simulink model "SIL_block"  (R2021b)
settings: Solver=FixedStepAuto  StartTime=0.0  StopTime=5  FixedStep=0.07  RelTol=1e-3
libraries: pil_lib x1
settings Model: Creator=Admin  LastModifiedBy=Admin
settings SolverCC: AlgebraicLoopSolver=TrustRegion
settings OptimizationCC: DefaultParameterBehavior=Inlined  EnhancedBackFolding=on  PassReuseOutputArgsThreshold=0  OptimizeBlockOrder=speed  DifferentSizesBufferReuse=on  OptimizationCustomize=off
settings DebuggingCC: ParameterTunabilityLossMsg=error  SFUnexpectedBacktrackingDiag=warning  SFNoUnconditionalDefaultTransitionDiag=warning  SFMachineParentedDataDiag=warning
settings SFSimCC: MATLABDynamicMemAlloc=off
settings RTWCC: GenCodeOnly=on  GenerateReport=on  BuildConfiguration=Debug  LaunchReport=on  CheckMdlBeforeBuild=Warning
settings CodeAppCC: ForceParamTrailComments=on  OperatorAnnotations=on  EnableCustomComments=on
settings ConfigComp: CovEnable=on  CovScope=Subsystem  RecordCoverage=on  CovPath=Subsystem/PID Controller1  CovMetricSettings=we  PLC_TargetIDE=codesys23  PLC_MultiTBSigbuilderTimeRange=off  PLC_InlineEnumCastFunction=off

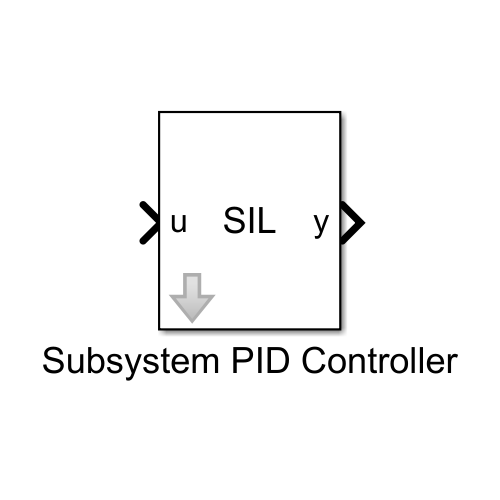
[thumbnail: Simulink's stored preview of the top-level diagram]
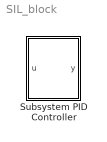
== system SIL_block ==
  Subsystem PID Controller : Subsystem  DialogController=pil_create_dialog  LoadFcn=|
      | try
      |    if ~strcmp(rtw.pil.getPILVersion, '9.11 (R2021b)_15')
      |       set_param(gcb, 'DialogController', '');
      |       set_param(gcb, 'DialogControllerArgs', '');
      |    end
      | catch e
      |       set_param(gcb, 'DialogController', '');
      |       set_param(gcb, 'DialogControllerArgs', '');
      | end
      mask help: PIL:pil:XILBlockMaskDesc
      mask Display: disp('SIL');

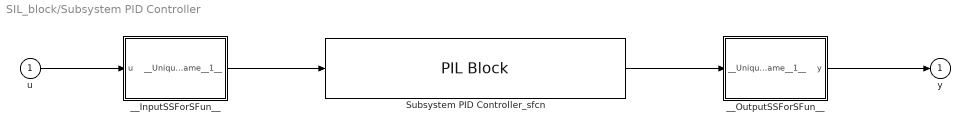
== system SIL_block/Subsystem PID Controller ==
  u : Inport
  Subsystem PID Controller_sfcn : pil_lib/PIL Block  SimulationMode=SIL  IsTopModelPIL=off  CodeDir=Subsystem_ert_rtw  AnchorDir=C:\Users\Admin\Documents\OneDrive\Рабочий стол\ПСвСМ 2022\Лекция1_23_PROGRAM  ConfigName=Software-in-the-Loop (SIL)  XrelIsTopModelCode=on  XrelIsReusable=off  XrelDWorkNames={}  XrelDWorkTypes={}  XrelModelArgVals={}  XrelOrderedParamNames={}
      settings: SourceProductBaseCode=RT
  __InputSSForSFun__ : Subsystem
  __OutputSSForSFun__ : Subsystem
  y : Outport
  wires:
  u/1 -> __InputSSForSFun__/1(u)
  __InputSSForSFun__/1(__UniqueOutportName__1__) -> Subsystem PID Controller_sfcn/1
  Subsystem PID Controller_sfcn/1 -> __OutputSSForSFun__/1(__UniqueInportName__1__)
  __OutputSSForSFun__/1(y) -> y/1

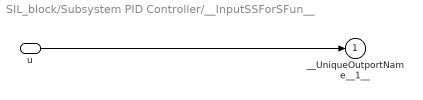
== system SIL_block/Subsystem PID Controller/__InputSSForSFun__ ==
  u : Inport
  __UniqueOutportName__1__ : Outport
  wires:
  u/1 -> __UniqueOutportName__1__/1

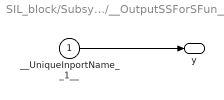
== system SIL_block/Subsystem PID Controller/__OutputSSForSFun__ ==
  __UniqueInportName__1__ : Inport
  y : Outport
  wires:
  __UniqueInportName__1__/1 -> y/1
